simulink model "Plant_completo_orig_forlinearization"  (R2023a)
settings: Solver=ode45  StartTime=0.0  StopTime=100  RelTol=1e-2  EnableMultiTasking=on
values from neighbouring files (symbols this model uses):
  alfa = [alfaa alfab alfac alfad alfae alfaf]    [ChemBenchData.m]    (also in dati.m)
  F0A = 100    [ChemBenchData.m]    (also in dati.m)
  F0B = 0.5    [ChemBenchData.m]    (also in dati.m)
  F0E = 99.5    [ChemBenchData.m]    (also in dati.m)
  H1 = [Hr1;He1*ones(Ne1,1);Hf1;Ha1*ones(Na1,1);Hc1]    [ChemBenchData.m]    (also in dati.m)
  H2 = [Hr2;He2*ones(Ne2,1);Hf2;Ha2*ones(Na2,1);Hc2]    [ChemBenchData.m]    (also in dati.m)
  H3 = [Hr3;He3*ones(Ne3,1);Hf3;Ha3*ones(Na3,1);Hc3]    [ChemBenchData.m]    (also in dati.m)
  k1 = 10    [ChemBenchData.m]    (also in dati.m)
  k2 = 50    [ChemBenchData.m]    (also in dati.m)
  N1 = Na1+Ne1+3    (= 19)    [ChemBenchData.m]    (also in dati.m = 9)
  N2 = Na2+Ne2+3    (= 19)    [ChemBenchData.m]    (also in dati.m = 9)
  N3 = Na3+Ne3+3    (= 19)    [ChemBenchData.m]    (also in dati.m = 9)
  Na1 = 8    [ChemBenchData.m]    (also in dati.m = 3)
  Na2 = 8    [ChemBenchData.m]    (also in dati.m = 3)
  Na3 = 8    [ChemBenchData.m]    (also in dati.m = 3)
  Ne1 = 8    [ChemBenchData.m]    (also in dati.m = 3)
  Ne2 = 8    [ChemBenchData.m]    (also in dati.m = 3)
  Ne3 = 8    [ChemBenchData.m]    (also in dati.m = 3)
  R1 = 330    [ChemBenchData.m]    (also in dati.m = 400)
  R2 = 283    [ChemBenchData.m]    (also in dati.m = 375)
  R3 = 141    [ChemBenchData.m]    (also in dati.m = 272)
  V1 = 330+80    (= 410)    [ChemBenchData.m]    (also in dati.m)
  V2 = 385    [ChemBenchData.m]    (also in dati.m = 405)
  V3 = 282    [ChemBenchData.m]    (also in dati.m)
  VR1 = 1000    [ChemBenchData.m]    (also in dati.m)
  VR2 = 850    [ChemBenchData.m]    (also in dati.m)
  x1a = zeros(N1,1)    [ChemBenchData.m]    (also in dati.m)
  x1b = zeros(N1,1)    [ChemBenchData.m]    (also in dati.m)
  x1c = zeros(N1,1)    [ChemBenchData.m]    (also in dati.m)
  x2a = zeros(N2,1)    [ChemBenchData.m]    (also in dati.m)
  x2b = zeros(N2,1)    [ChemBenchData.m]    (also in dati.m)
  x2c = zeros(N2,1)    [ChemBenchData.m]    (also in dati.m)
  x3a = zeros(N3,1)    [ChemBenchData.m]    (also in dati.m)
  x3b = zeros(N3,1)    [ChemBenchData.m]    (also in dati.m)
  x3c = zeros(N3,1)    [ChemBenchData.m]    (also in dati.m)
  xD3_a = 0.    (= 0)    [ChemBenchData.m]    (also in dati.m)
  xD3_c = 0.0036    [ChemBenchData.m]    (also in dati.m)
  xD3_d = 0.2817    [ChemBenchData.m]    (also in dati.m)
  z0A_a = 1    [ChemBenchData.m]    (also in dati.m)
  z0A_b = 0    [ChemBenchData.m]    (also in dati.m)
  z0A_c = 0    [ChemBenchData.m]    (also in dati.m)
  z0A_d = 0    [ChemBenchData.m]    (also in dati.m)
  z0B_a = 0    [ChemBenchData.m]    (also in dati.m)
  z0B_b = 1    [ChemBenchData.m]    (also in dati.m)
  z0B_c = 0    [ChemBenchData.m]    (also in dati.m)
  z0B_d = 0    [ChemBenchData.m]    (also in dati.m)
  z0E_b = 0    [ChemBenchData.m]    (also in dati.m)
  z0E_d = 0    [ChemBenchData.m]    (also in dati.m)
  z0E_e = 1    [ChemBenchData.m]    (also in dati.m)
  z0E_f = 0    [ChemBenchData.m]    (also in dati.m)
  z1a = 0.184    [ChemBenchData.m]    (also in R1_stati.m = u(1); dati.m)
  z1b = 0.0544    [ChemBenchData.m]    (also in R1_stati.m = u(2); dati.m)
  z1c = 0.3255    [ChemBenchData.m]    (also in R1_stati.m = u(3); dati.m)
  z1d = 0.4361    [ChemBenchData.m]    (also in R1_stati.m = u(4); dati.m)
  z2b = 0.4455    [ChemBenchData.m]    (also in dati.m)
  z2d = 0.0514    [ChemBenchData.m]    (also in dati.m)
  z2e = 0.0411    [ChemBenchData.m]    (also in dati.m)
  z2f = 0.4455    [ChemBenchData.m]    (also in dati.m)
  z3b = 0.4666    [ChemBenchData.m]    (also in dati.m)
  z3d = 0.0523    [ChemBenchData.m]    (also in dati.m)
  z3e = 0.0032    [ChemBenchData.m]    (also in dati.m)
  z3f = 0.4666    [ChemBenchData.m]    (also in dati.m)
undefined symbols (not defined in the file or in its folder): colonna1, colonna2, colonna3, R1_portata, R1_stati, R2_portata, R2_stati, R3_portata, R3_stati, somma
libraries: simulink x1
settings Model: Creator=scattolini  LastModifiedBy=laura
settings SolverCC: AlgebraicLoopSolver=TrustRegion
settings DataIOCC: LimitDataPoints=on  SaveFormat=Array  SignalLoggingSaveFormat=ModelDataLogs  ReturnWorkspaceOutputs=off
settings OptimizationCC: BlockReduction=off  DefaultParameterBehavior=Inlined  InlineInvariantSignals=on  BufferReuse=off  ExpressionDepthLimit=2147483647  InitFltsAndDblsToZero=on  LifeSpan=inf
settings DebuggingCC: SaveWithParameterizedLinksMsg=none  UnderspecifiedInitializationDetection=Classic  MergeDetectMultiDrivingBlocksExec=none  SignalResolutionControl=TryResolveAllWithWarning  SolverPrmCheckMsg=warning  MultiTaskDSMMsg=warning  MultiTaskCondExecSysMsg=none  FcnCallInpInsideContextMsg=warning  UnconnectedInputMsg=warning  UnconnectedOutputMsg=warning  UnconnectedLineMsg=warning  StateNameClashWarn=warning  SFUnexpectedBacktrackingDiag=warning  SFNoUnconditionalDefaultTransitionDiag=warning  SFExecutionAtInitializationDiag=none  ArithmeticOperatorsInVariantConditions=warning
settings HardwareCC: ProdBitPerPointer=32  ProdBitPerSizeT=32  ProdBitPerPtrDiffT=32  ProdLargestAtomicFloat=None  ProdIntDivRoundTo=Undefined  ProdEndianess=Unspecified  ProdWordSize=32  ProdHWDeviceType=32-bit Generic
settings ModelReferenceCC: EnableRefExpFcnMdlSchedulingChecks=on  PropagateSignalLabelsOutOfModel=off
settings RTWCC: DLArmComputeVersion=19.05
settings CodeAppCC: StateflowObjectComments=on
settings GRTTargetCC: TargetFcnLib=ansi_tfl_tmw.mat  TargetLangStandard=C89/C90 (ANSI)  CombineOutputUpdateFcns=off  GRTInterface=on
settings ConfigComp: CovMetricSettings=dw  CovSaveCumulativeToWorkspaceVar=on  CovSaveSingleToWorkspaceVar=on

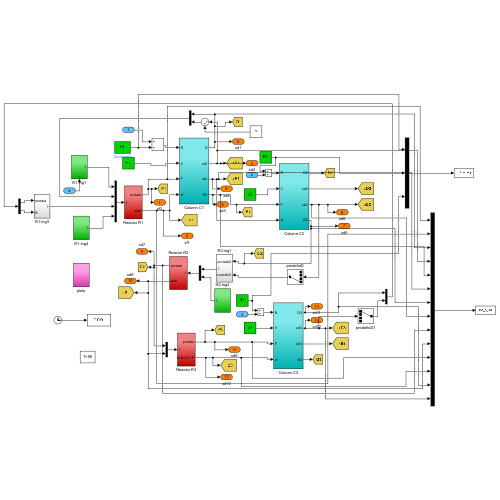
[thumbnail: Simulink's stored preview of the top-level diagram]
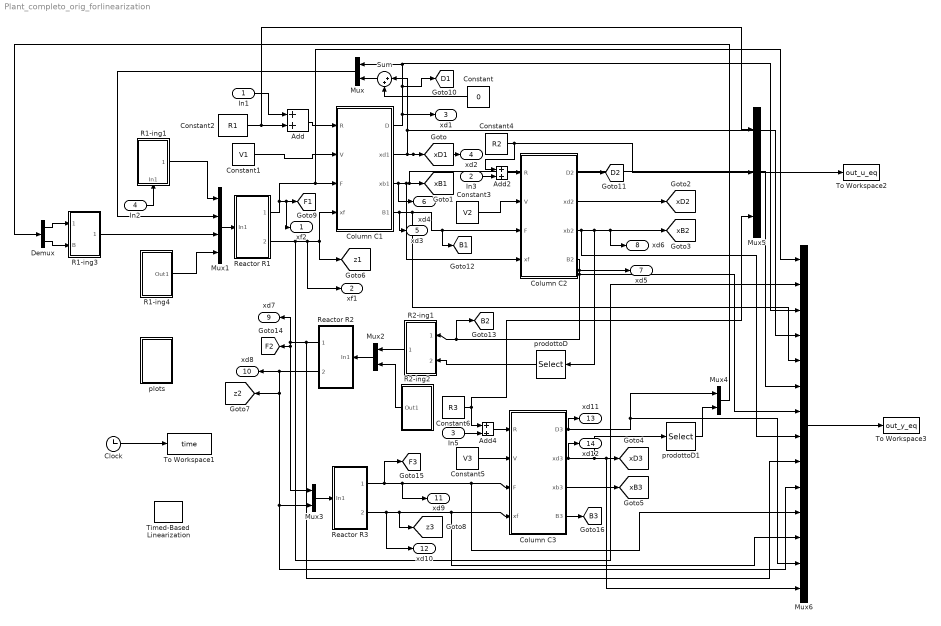
== system Plant_completo_orig_forlinearization ==
  In1 : Inport
  In3 : Inport  Port=2
  In5 : Inport  Port=3
  In2 : Inport  Port=4
  Add : Sum
  Add2 : Sum
  Add4 : Sum
  Clock : Clock
  Column C1 : Subsystem
  Column C2 : Subsystem
  Column C3 : Subsystem
  Constant : Constant  Value=0
  Constant1 : Constant  Value=V1
  Constant2 : Constant  Value=R1
  Constant3 : Constant  Value=V2
  Constant4 : Constant  Value=R2
  Constant5 : Constant  Value=V3
  Constant6 : Constant  Value=R3
  Demux : Demux  Outputs=2
  Mux{,2..4} (4 alike) : Mux  Inputs=2
  Mux1 : Mux
  Mux5 : Mux  Inputs=3
  Mux6 : Mux  Inputs=14
  R1-ing1 : Subsystem
      settings: PortSchema="{\"entries\":[{\"content\":{\"sides\":[{\"content\":{},\"type\":\"ConnectorPlacement.EquallySpacedRectSide\",\"uuid\":\"2596f0e2-5755-4d6d-8ea6-258356428fbb\"},{\"content\":{\"connectorIds\":[\"Out1\"],\"side\":\"RIGHT\"},\"type\":\"ConnectorPlacement.EquallySpacedRectSide\",\"uuid\":\"94d46858-4830-4a6d-8661-aa93a1271d75\"},{\"content\":{\"side\":\"TOP\"},\"type\":\"ConnectorPlacement.EquallySpacedRectSide\",\"uuid\":\"cb66ff0a-24ad-4581-b318-24253491df81\"},{\"content\":{\"connectorIds\":[\"In1\"],\"side\":\"BOTTOM\"},\"type\":\"ConnectorPlacement.EquallySpacedRectSide\",\"uuid\":\"dffee1b5-3318-48a5-a504-ed15a4323ec4\"}]},\"type\":\"ConnectorPlacement.EquallySpacedConnector\",\"uuid\":\"2dd9660c-c0b8-471f-9483-861c836841d9\"}],\"packageUris\":[\"http://schema.mathworks.com/mf0/Connector/R2020b\"],\"version\":\"1.0\"}"
  R1-ing3 : Subsystem
  R1-ing4 : Subsystem
  R2-ing1 : Subsystem
  R2-ing2 : Subsystem
  Reactor R1 : Subsystem
  Reactor R2 : Subsystem
  Reactor R3 : Subsystem
  Sum : Sum  Inputs=|++
  Timed-Based Linearization : simulink/Model-Wide Utilities/Timed-Based Linearization  LinearizationTime=99  SampleTime=0
  To Workspace1 : ToWorkspace  VariableName=time  SampleTime=-1
  To Workspace2 : ToWorkspace  VariableName=out_u_eq  SampleTime=1
  To Workspace3 : ToWorkspace  VariableName=out_y_eq  SampleTime=1
  plots : Subsystem
  prodottoD : Selector  InputPortWidth=4  IndexOptions=Index vector (dialog)  Indices=4  OutputSizes=1
  prodottoD1 : Selector  InputPortWidth=4  IndexOptions=Index vector (dialog)  Indices=1  OutputSizes=1
  xf2 : Outport
  xf1 : Outport  Port=2
  xd1 : Outport  Port=3
  xd2 : Outport  Port=4
  xd3 : Outport  Port=5
  xd4 : Outport  Port=6
  xd5 : Outport  Port=7
  xd6 : Outport  Port=8
  xd7 : Outport  Port=9
  xd8 : Outport  Port=10
  xd9 : Outport  Port=11
  xd10 : Outport  Port=12
  xd11 : Outport  Port=13
  xd12 : Outport  Port=14
  tag scope: B1=global, B2=global, B3=global, D1=global, D2=global, F1=global, F2=global, F3=global, xB1=global, xB2=global, xB3=global, xD1=global, xD2=global, xD3=global, z1=global, z2=global, z3=global
  wires:
  R1-ing1/1(Out1) -> Mux1/1
  R1-ing3/1(Out1) -> Mux1/3
  R1-ing4/1(Out1) -> Mux1/4
  Mux1/1 -> Reactor R1/1(In1)
  Column C1/3(xb1) -> xd4/1, Mux6/6, [xB1], Column C2/4(xf)
  Column C1/2(xd1) -> Sum/1, Mux6/4, xd2/1, [xD1]
  Column C1/1(D) -> xd1/1, Mux6/3, Mux/1, [D1]
  Mux/1 -> Mux1/2
  Column C1/4(B1) -> xd3/1, Mux6/5, Column C2/3(F), [B1]
  Column C2/3(xb2) -> Mux6/8, prodottoD/1, xd6/1, [xB2]
  Column C2/4(B2) -> xd5/1, Mux6/7, R2-ing1/1(portataD), [B2]
  prodottoD/1 -> R2-ing1/2(prodottoD)
  Mux2/1 -> Reactor R2/1(In1)
  R2-ing1/1(Out1) -> Mux2/1
  R2-ing2/1(Out1) -> Mux2/2
  Reactor R1/1(portata) -> Mux6/1, Column C1/3(F), xf2/1, [F1]
  Reactor R1/2(stati) -> Mux6/2, xf1/1, Column C1/4(xf), [z1]
  Reactor R2/2(stati) -> xd8/1, Mux6/10, Mux3/2, [z2]
  Reactor R2/1(portata) -> xd7/1, Mux3/1, [F2], Mux6/9
  Mux3/1 -> Reactor R3/1(In1)
  Reactor R3/1(portata) -> xd9/1, Mux6/11, Column C3/3(F), [F3]
  Reactor R3/2(stati B-D-E-F) -> xd10/1, Mux6/12, Column C3/4(xf), [z3]
  Column C3/3(xb3) -> [xB3]
  Column C3/2(xd3) -> xd12/1, Mux6/14, [xD3], prodottoD1/1
  Column C2/2(xd2) -> [xD2]
  Column C2/1(D2) -> [D2]
  prodottoD1/1 -> Mux4/2
  Column C3/1(D3) -> xd11/1, Mux4/1, Mux6/13
  Mux4/1 -> Demux/1
  Demux/1 -> R1-ing3/1(portata)
  Demux/2 -> R1-ing3/2(B)
  Clock/1 -> To Workspace1/1
  In1/1 -> Add/1
  Add/1 -> Column C1/1(R)
  Constant1/1 -> Column C1/2(V)
  Add2/1 -> Column C2/1(R)
  Constant4/1 -> Mux5/2, Add2/1
  Constant3/1 -> Column C2/2(V)
  In3/1 -> Add2/2
  Constant6/1 -> Mux5/3, Add4/1
  Constant5/1 -> Column C3/2(V)
  In5/1 -> Add4/2
  Column C3/4(B3) -> [B3]
  Add4/1 -> Column C3/1(R)
  Mux5/1 -> To Workspace2/1
  Mux6/1 -> To Workspace3/1
  Constant2/1 -> Mux5/1, Add/2
  In2/1 -> R1-ing1/1(In1)
  Sum/1 -> Mux/2
  Constant/1 -> Sum/2

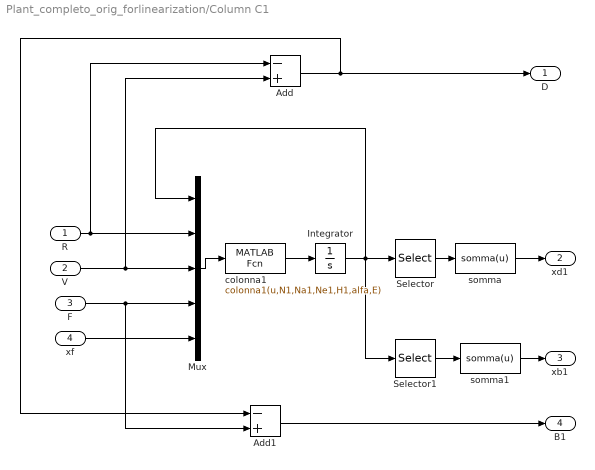
== system Plant_completo_orig_forlinearization/Column C1 ==
  R : Inport
  V : Inport  Port=2
  F : Inport  Port=3
  xf : Inport  Port=4
  Add : Sum  Inputs=-+
  Add1 : Sum  Inputs=-+
  Integrator : Integrator  InitialCondition=[x1a;x1b;x1c]
  Mux : Mux  Inputs=5
  Selector : Selector  InputPortWidth=N1*3  IndexOptions=Index vector (dialog)  Indices=[N1 2*N1 3*N1]  OutputSizes=1
  Selector1 : Selector  InputPortWidth=N1*3  IndexOptions=Index vector (dialog)  Indices=[1 N1+1 2*N1+1]  OutputSizes=1
  colonna1 : MATLABFcn  MATLABFcn=colonna1(u,N1,Na1,Ne1,H1,alfa,E)  OutputDimensions=N1*3
  somma : MATLABFcn  MATLABFcn=somma(u)  OutputDimensions=4
  somma1 : MATLABFcn  MATLABFcn=somma(u)  OutputDimensions=4
  D : Outport
  xd1 : Outport  Port=2
  xb1 : Outport  Port=3
  B1 : Outport  Port=4
  wires:
  Mux/1 -> colonna1/1
  colonna1/1 -> Integrator/1
  Integrator/1 -> Selector/1, Mux/1, Selector1/1
  R/1 -> Mux/2, Add/1
  V/1 -> Mux/3, Add/2
  F/1 -> Mux/4, Add1/2
  xf/1 -> Mux/5
  Selector/1 -> somma/1
  somma/1 -> xd1/1
  Selector1/1 -> somma1/1
  somma1/1 -> xb1/1
  Add/1 -> D/1, Add1/1
  Add1/1 -> B1/1

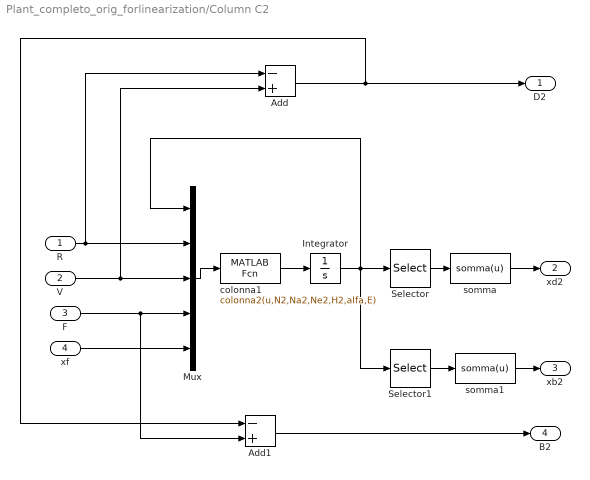
== system Plant_completo_orig_forlinearization/Column C2 ==
  R : Inport
  V : Inport  Port=2
  F : Inport  Port=3
  xf : Inport  Port=4
  Add : Sum  Inputs=-+
  Add1 : Sum  Inputs=-+
  Integrator : Integrator  InitialCondition=[x2a;x2b;x2c]
  Mux : Mux  Inputs=5
  Selector : Selector  InputPortWidth=N2*3  IndexOptions=Index vector (dialog)  Indices=[N2 2*N2 3*N2]  OutputSizes=1
  Selector1 : Selector  InputPortWidth=N2*3  IndexOptions=Index vector (dialog)  Indices=[1 N2+1 2*N2+1]  OutputSizes=1
  colonna1 : MATLABFcn  MATLABFcn=colonna2(u,N2,Na2,Ne2,H2,alfa,E)  OutputDimensions=N2*3
  somma : MATLABFcn  MATLABFcn=somma(u)  OutputDimensions=4
  somma1 : MATLABFcn  MATLABFcn=somma(u)  OutputDimensions=4
  D2 : Outport
  xd2 : Outport  Port=2
  xb2 : Outport  Port=3
  B2 : Outport  Port=4
  wires:
  Mux/1 -> colonna1/1
  colonna1/1 -> Integrator/1
  Integrator/1 -> Selector/1, Mux/1, Selector1/1
  R/1 -> Mux/2, Add/1
  V/1 -> Mux/3, Add/2
  F/1 -> Mux/4, Add1/2
  xf/1 -> Mux/5
  Selector/1 -> somma/1
  somma/1 -> xd2/1
  Selector1/1 -> somma1/1
  somma1/1 -> xb2/1
  Add/1 -> D2/1, Add1/1
  Add1/1 -> B2/1

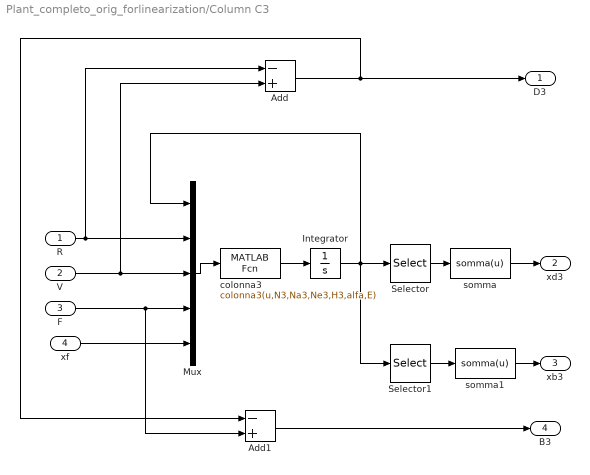
== system Plant_completo_orig_forlinearization/Column C3 ==
  R : Inport
  V : Inport  Port=2
  F : Inport  Port=3
  xf : Inport  Port=4
  Add : Sum  Inputs=-+
  Add1 : Sum  Inputs=-+
  Integrator : Integrator  InitialCondition=[x3a;x3b;x3c]
  Mux : Mux  Inputs=5
  Selector : Selector  InputPortWidth=N3*3  IndexOptions=Index vector (dialog)  Indices=[N3 2*N3 3*N3]  OutputSizes=1
  Selector1 : Selector  InputPortWidth=N3*3  IndexOptions=Index vector (dialog)  Indices=[1 N3+1 2*N3+1]  OutputSizes=1
  colonna3 : MATLABFcn  MATLABFcn=colonna3(u,N3,Na3,Ne3,H3,alfa,E)  OutputDimensions=N3*3
  somma : MATLABFcn  MATLABFcn=somma(u)  OutputDimensions=4
  somma1 : MATLABFcn  MATLABFcn=somma(u)  OutputDimensions=4
  D3 : Outport
  xd3 : Outport  Port=2
  xb3 : Outport  Port=3
  B3 : Outport  Port=4
  wires:
  Mux/1 -> colonna3/1
  colonna3/1 -> Integrator/1
  Integrator/1 -> Selector/1, Mux/1, Selector1/1
  R/1 -> Mux/2, Add/1
  V/1 -> Mux/3, Add/2
  F/1 -> Mux/4, Add1/2
  xf/1 -> Mux/5
  Selector/1 -> somma/1
  somma/1 -> xd3/1
  Selector1/1 -> somma1/1
  somma1/1 -> xb3/1
  Add/1 -> D3/1, Add1/1
  Add1/1 -> B3/1

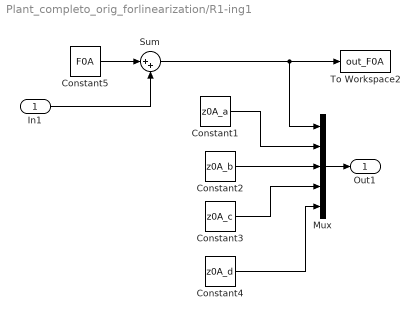
== system Plant_completo_orig_forlinearization/R1-ing1 ==
  In1 : Inport
  Constant1 : Constant  Value=z0A_a
  Constant2 : Constant  Value=z0A_b
  Constant3 : Constant  Value=z0A_c
  Constant4 : Constant  Value=z0A_d
  Constant5 : Constant  Value=F0A
  Mux : Mux  Inputs=5
  Sum : Sum  Inputs=|++
  To Workspace2 : ToWorkspace  VariableName=out_F0A  SampleTime=1
  Out1 : Outport
  wires:
  Constant1/1 -> Mux/2
  Constant2/1 -> Mux/3
  Constant3/1 -> Mux/4
  Constant4/1 -> Mux/5
  Mux/1 -> Out1/1
  Constant5/1 -> Sum/1
  Sum/1 -> Mux/1, To Workspace2/1
  In1/1 -> Sum/2

== system Plant_completo_orig_forlinearization/R1-ing3 ==
  portata : Inport
  B : Inport  Port=2
  Constant1 : Constant  Value=xD3_a
  Constant3 : Constant  Value=xD3_c
  Constant4 : Constant  Value=xD3_d
  Mux : Mux  Inputs=5
  Out1 : Outport
  wires:
  portata/1 -> Mux/1
  Constant1/1 -> Mux/2
  B/1 -> Mux/3
  Constant3/1 -> Mux/4
  Constant4/1 -> Mux/5
  Mux/1 -> Out1/1

== system Plant_completo_orig_forlinearization/R1-ing4 ==
  Constant : Constant  Value=F0B
  Constant1 : Constant  Value=z0B_a
  Constant2 : Constant  Value=z0B_b
  Constant3 : Constant  Value=z0B_c
  Constant4 : Constant  Value=z0B_d
  Mux : Mux  Inputs=5
  Out1 : Outport
  wires:
  Constant/1 -> Mux/1
  Constant1/1 -> Mux/2
  Constant2/1 -> Mux/3
  Constant3/1 -> Mux/4
  Constant4/1 -> Mux/5
  Mux/1 -> Out1/1

== system Plant_completo_orig_forlinearization/R2-ing1 ==
  portataD : Inport
  prodottoD : Inport  Port=2
  Constant2 : Constant  Value=0
  Constant3 : Constant  Value=0
  Constant4 : Constant  Value=0
  Mux : Mux  Inputs=5
  Out1 : Outport
  wires:
  portataD/1 -> Mux/1
  prodottoD/1 -> Mux/2
  Constant2/1 -> Mux/3
  Constant3/1 -> Mux/4
  Constant4/1 -> Mux/5
  Mux/1 -> Out1/1

== system Plant_completo_orig_forlinearization/R2-ing2 ==
  Constant : Constant  Value=F0E
  Constant1 : Constant  Value=z0E_d
  Constant2 : Constant  Value=z0E_e
  Constant3 : Constant  Value=z0E_f
  Constant4 : Constant  Value=z0E_b
  Mux : Mux  Inputs=5
  Out1 : Outport
  wires:
  Constant/1 -> Mux/1
  Constant1/1 -> Mux/2
  Constant2/1 -> Mux/3
  Constant3/1 -> Mux/4
  Constant4/1 -> Mux/5
  Mux/1 -> Out1/1

== system Plant_completo_orig_forlinearization/Reactor R1 ==
  In1 : Inport
  Integrator1 : Integrator  InitialCondition=[z1a z1b z1c z1d]
  Mux2 : Mux  Inputs=2
  R1_portata : MATLABFcn  MATLABFcn=R1_portata(u)
  R1_stati : MATLABFcn  MATLABFcn=R1_stati(u,k1,VR1)  OutputDimensions=4
  portata : Outport
  stati : Outport  Port=2
  wires:
  In1/1 -> Mux2/2, R1_portata/1
  R1_stati/1 -> Integrator1/1
  Mux2/1 -> R1_stati/1
  Integrator1/1 -> Mux2/1, stati/1
  R1_portata/1 -> portata/1

== system Plant_completo_orig_forlinearization/Reactor R2 ==
  In1 : Inport
  Integrator1 : Integrator  InitialCondition=[z2d z2e z2f z2b]
  Mux2 : Mux  Inputs=2
  R2_portata : MATLABFcn  MATLABFcn=R2_portata(u)
  R2_stati : MATLABFcn  MATLABFcn=R2_stati(u,k2,VR2)  OutputDimensions=4
  portata : Outport
  stati : Outport  Port=2
  wires:
  In1/1 -> Mux2/2, R2_portata/1
  R2_stati/1 -> Integrator1/1
  Mux2/1 -> R2_stati/1
  Integrator1/1 -> Mux2/1, stati/1
  R2_portata/1 -> portata/1

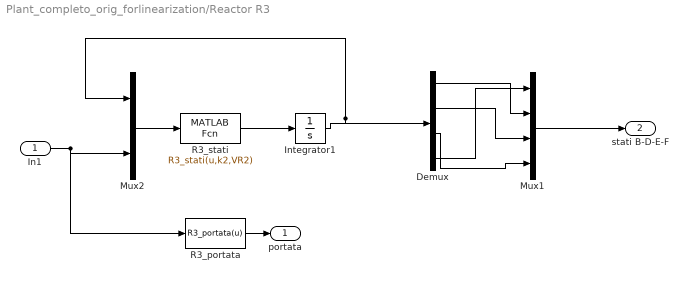
== system Plant_completo_orig_forlinearization/Reactor R3 ==
  In1 : Inport
  Demux : Demux
  Integrator1 : Integrator  InitialCondition=[z3d z3e z3f z3b]
  Mux1 : Mux
  Mux2 : Mux  Inputs=2
  R3_portata : MATLABFcn  MATLABFcn=R3_portata(u)
  R3_stati : MATLABFcn  MATLABFcn=R3_stati(u,k2,VR2)  OutputDimensions=4
  portata : Outport
  stati B-D-E-F : Outport  Port=2
  wires:
  In1/1 -> Mux2/2, R3_portata/1
  R3_stati/1 -> Integrator1/1
  Mux2/1 -> R3_stati/1
  Integrator1/1 -> Mux2/1, Demux/1
  R3_portata/1 -> portata/1
  Demux/4 -> Mux1/1
  Demux/1 -> Mux1/2
  Demux/2 -> Mux1/3
  Demux/3 -> Mux1/4
  Mux1/1 -> stati B-D-E-F/1

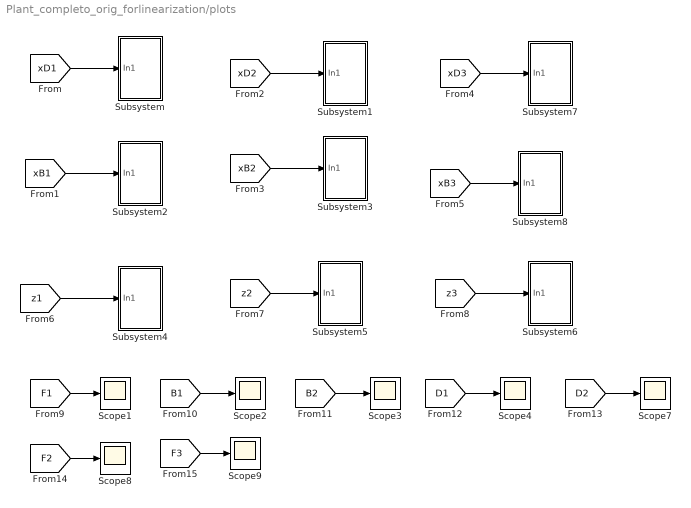
== system Plant_completo_orig_forlinearization/plots ==
  Scope{1..4,7..9} (7 alike) : Scope
  Subsystem : Subsystem
  Subsystem1 : Subsystem
  Subsystem2 : Subsystem
  Subsystem3 : Subsystem
  Subsystem4 : Subsystem
  Subsystem5 : Subsystem
  Subsystem6 : Subsystem
  Subsystem7 : Subsystem
  Subsystem8 : Subsystem
  wires:
  [z2] -> Subsystem5/1(In1)
  [xD1] -> Subsystem/1(In1)
  [xD2] -> Subsystem1/1(In1)
  [xB1] -> Subsystem2/1(In1)
  [xB2] -> Subsystem3/1(In1)
  [z1] -> Subsystem4/1(In1)
  [z3] -> Subsystem6/1(In1)
  [F1] -> Scope1/1
  [B1] -> Scope2/1
  [B2] -> Scope3/1
  [D1] -> Scope4/1
  [D2] -> Scope7/1
  [F2] -> Scope8/1
  [F3] -> Scope9/1
  [xD3] -> Subsystem7/1(In1)
  [xB3] -> Subsystem8/1(In1)

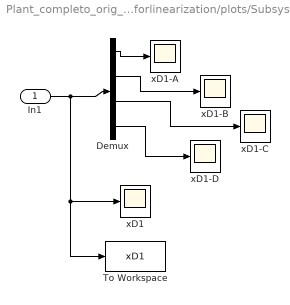
== system Plant_completo_orig_forlinearization/plots/Subsystem ==
  In1 : Inport
  Demux : Demux
  To Workspace : ToWorkspace  VariableName=xD1  SampleTime=-1
  xD1 : Scope
  xD1-A : Scope
  xD1-B : Scope
  xD1-C : Scope
  xD1-D : Scope
  wires:
  In1/1 -> xD1/1, To Workspace/1, Demux/1
  Demux/1 -> xD1-A/1
  Demux/2 -> xD1-B/1
  Demux/3 -> xD1-C/1
  Demux/4 -> xD1-D/1

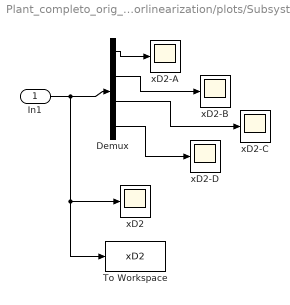
== system Plant_completo_orig_forlinearization/plots/Subsystem1 ==
  In1 : Inport
  Demux : Demux
  To Workspace : ToWorkspace  VariableName=xD2  SampleTime=-1
  xD2 : Scope
  xD2-A : Scope
  xD2-B : Scope
  xD2-C : Scope
  xD2-D : Scope
  wires:
  In1/1 -> xD2/1, To Workspace/1, Demux/1
  Demux/1 -> xD2-A/1
  Demux/2 -> xD2-B/1
  Demux/3 -> xD2-C/1
  Demux/4 -> xD2-D/1

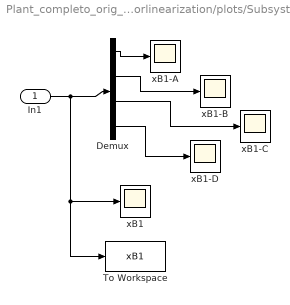
== system Plant_completo_orig_forlinearization/plots/Subsystem2 ==
  In1 : Inport
  Demux : Demux
  To Workspace : ToWorkspace  VariableName=xB1  SampleTime=-1
  xB1 : Scope
  xB1-A : Scope
  xB1-B : Scope
  xB1-C : Scope
  xB1-D : Scope
  wires:
  In1/1 -> xB1/1, To Workspace/1, Demux/1
  Demux/1 -> xB1-A/1
  Demux/2 -> xB1-B/1
  Demux/3 -> xB1-C/1
  Demux/4 -> xB1-D/1

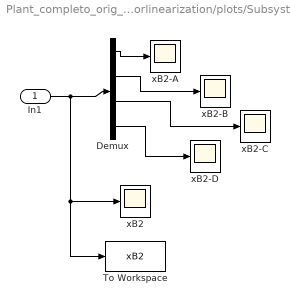
== system Plant_completo_orig_forlinearization/plots/Subsystem3 ==
  In1 : Inport
  Demux : Demux
  To Workspace : ToWorkspace  VariableName=xB2  SampleTime=-1
  xB2 : Scope
  xB2-A : Scope
  xB2-B : Scope
  xB2-C : Scope
  xB2-D : Scope
  wires:
  In1/1 -> xB2/1, To Workspace/1, Demux/1
  Demux/1 -> xB2-A/1
  Demux/2 -> xB2-B/1
  Demux/3 -> xB2-C/1
  Demux/4 -> xB2-D/1

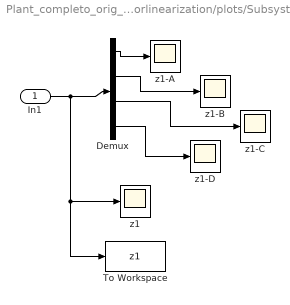
== system Plant_completo_orig_forlinearization/plots/Subsystem4 ==
  In1 : Inport
  Demux : Demux
  To Workspace : ToWorkspace  VariableName=z1  SampleTime=-1
  z1 : Scope
  z1-A : Scope
  z1-B : Scope
  z1-C : Scope
  z1-D : Scope
  wires:
  In1/1 -> z1/1, To Workspace/1, Demux/1
  Demux/1 -> z1-A/1
  Demux/2 -> z1-B/1
  Demux/3 -> z1-C/1
  Demux/4 -> z1-D/1

== system Plant_completo_orig_forlinearization/plots/Subsystem5 ==
  In1 : Inport
  Demux : Demux
  To Workspace : ToWorkspace  VariableName=z2  SampleTime=-1
  z1-D : Scope
  z2 : Scope
  z2-D : Scope
  z2-E : Scope
  z2-F : Scope
  wires:
  In1/1 -> z2/1, To Workspace/1, Demux/1
  Demux/1 -> z2-D/1
  Demux/2 -> z2-E/1
  Demux/3 -> z2-F/1
  Demux/4 -> z1-D/1

== system Plant_completo_orig_forlinearization/plots/Subsystem6 ==
  In1 : Inport
  Demux : Demux
  To Workspace : ToWorkspace  VariableName=z3  SampleTime=-1
  z3 : Scope
  z3-B1 : Scope
  z3-D : Scope
  z3-E : Scope
  z3-F : Scope
  wires:
  In1/1 -> z3/1, To Workspace/1, Demux/1
  Demux/1 -> z3-B1/1
  Demux/2 -> z3-D/1
  Demux/3 -> z3-E/1
  Demux/4 -> z3-F/1

== system Plant_completo_orig_forlinearization/plots/Subsystem7 ==
  In1 : Inport
  Demux : Demux
  To Workspace : ToWorkspace  VariableName=xD3  SampleTime=-1
  xD3 : Scope
  xD3-B : Scope
  xD3-D : Scope
  xD3-E : Scope
  xD3-F : Scope
  wires:
  In1/1 -> xD3/1, To Workspace/1, Demux/1
  Demux/1 -> xD3-B/1
  Demux/2 -> xD3-D/1
  Demux/3 -> xD3-E/1
  Demux/4 -> xD3-F/1

== system Plant_completo_orig_forlinearization/plots/Subsystem8 ==
  In1 : Inport
  Demux : Demux
  To Workspace : ToWorkspace  VariableName=xB3  SampleTime=-1
  xB3 : Scope
  xB3-B : Scope
  xB3-D : Scope
  xB3-E : Scope
  xB3-F : Scope
  wires:
  In1/1 -> xB3/1, To Workspace/1, Demux/1
  Demux/1 -> xB3-B/1
  Demux/2 -> xB3-D/1
  Demux/3 -> xB3-E/1
  Demux/4 -> xB3-F/1
